simulink model "discrete_nonlinear_model"  (R2024a)
settings: Solver=ode45  StartTime=0.0  StopTime=10  RelTol=1e-3  EnableMultiTasking=on
values from neighbouring files (symbols this model uses):
  m = calculate_model(p, T, tau_e)    [init.m]
  omega0 = 20    [init.m]
  reg = syn_regulator(m, 0.1, T)    [init.m]
  T = 0.00064    [init.m]
  tau_e = 0.005    [init.m]
settings Model: Creator=oleg  LastModifiedBy=olgatsybina
settings SolverCC: AlgebraicLoopSolver=TrustRegion
settings DataIOCC: LimitDataPoints=on  SaveFormat=Array  ReturnWorkspaceOutputs=off
settings OptimizationCC: LifeSpan=inf
settings DebuggingCC: SolverPrmCheckMsg=warning  UnconnectedInputMsg=warning  UnconnectedOutputMsg=warning  UnconnectedLineMsg=warning  SFUnexpectedBacktrackingDiag=warning  SFNoUnconditionalDefaultTransitionDiag=warning  SFExecutionAtInitializationDiag=none  ArithmeticOperatorsInVariantConditions=warning
settings HardwareCC: ProdBitPerPointer=32  ProdBitPerSizeT=32  ProdBitPerPtrDiffT=32  ProdLargestAtomicFloat=None  ProdIntDivRoundTo=Undefined  ProdEndianess=Unspecified  ProdWordSize=32  ProdHWDeviceType=32-bit Generic
settings ModelReferenceCC: EnableRefExpFcnMdlSchedulingChecks=on  PropagateSignalLabelsOutOfModel=off
settings SFSimCC: SimUseLocalCustomCode=off  CustomCodeUndefinedFunction=UseInterfaceOnly
settings RTWCC: RTWUseLocalCustomCode=off  GPUComputeCapability=3.5  DLArmComputeVersion=19.05
settings CodeAppCC: StateflowObjectComments=on
settings GRTTargetCC: TargetLangStandard=C89/C90 (ANSI)
settings ConfigComp: CovMetricSettings=dw  CovSaveCumulativeToWorkspaceVar=on  CovSaveSingleToWorkspaceVar=on  CovExternalEMLEnable=off  CovSFcnEnable=off

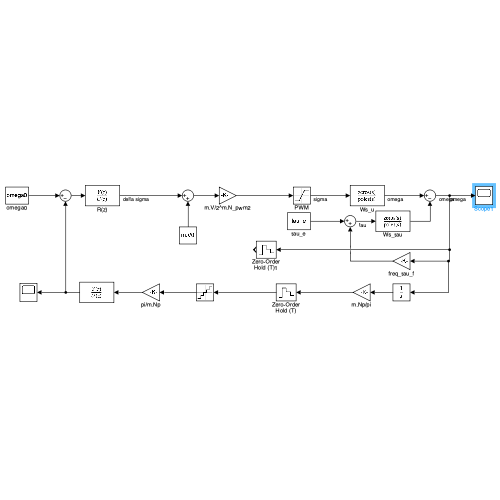
[thumbnail: Simulink's stored preview of the top-level diagram]
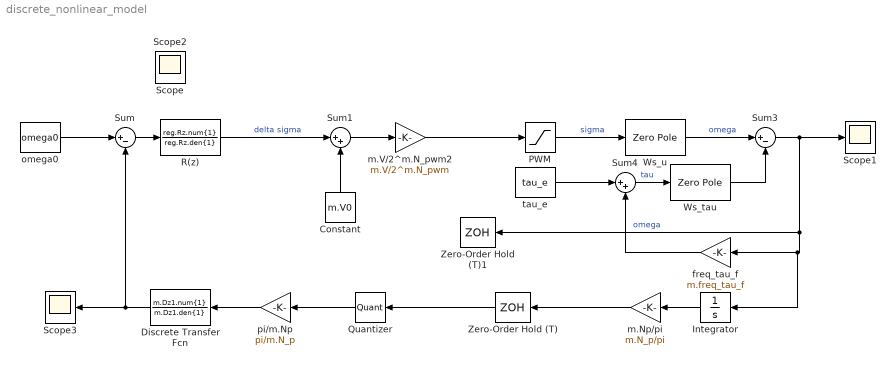
== system discrete_nonlinear_model ==
  Constant : Constant  Value=m.V0
  Discrete Transfer Fcn : DiscreteTransferFcn  Numerator=m.Dz1.num{1}  Denominator=m.Dz1.den{1}
  Integrator : Integrator
  PWM : Saturate  UpperLimit=m.V  LowerLimit=-m.V
  Quantizer : Quantizer  QuantizationInterval=1
  R(z) : DiscreteTransferFcn  Numerator=reg.Rz.num{1}  Denominator=reg.Rz.den{1}  SampleTime=T
  Scope{,1..3} (4 alike) : Scope
  Sum : Sum  Inputs=|+-
  Sum1 : Sum  Inputs=|++
  Sum3 : Sum  Inputs=|+-
  Sum4 : Sum  Inputs=|++
  Ws_tau : ZeroPole  Zeros=m.Ws_tau.Z{1}  Poles=m.Ws_tau.P{1}  Gain=m.Ws_tau.K
  Ws_u : ZeroPole  Zeros=m.Ws_u.Z{1}  Poles=m.Ws_u.P{1}  Gain=m.Ws_u.K
  Zero-Order Hold (T) : ZeroOrderHold  SampleTime=T
  Zero-Order Hold (T)1 : ZeroOrderHold  SampleTime=T
  freq_tau_f : Gain  Gain=m.freq_tau_f
  m.Np/pi : Gain  Gain=m.N_p/pi
  m.V/2^m.N_pwm2 : Gain  Gain=m.V/2^m.N_pwm
  omega0 : Constant  Value=omega0  SampleTime=T
  pi/m.Np : Gain  Gain=pi/m.N_p
  tau_e : Constant  Value=tau_e  SampleTime=T
  wires:
  omega0/1 -> Sum/1
  Sum/1 -> R(z)/1
  Zero-Order Hold (T)/1 -> Quantizer/1
  Sum3/1 -> Scope1/1, Zero-Order Hold (T)1/1, Integrator/1, freq_tau_f/1  "omega"
  freq_tau_f/1 -> Sum4/2
  Sum4/1 -> Ws_tau/1  "tau"
  tau_e/1 -> Sum4/1
  Ws_u/1 -> Sum3/1  "omega"
  Integrator/1 -> m.Np/pi/1
  m.Np/pi/1 -> Zero-Order Hold (T)/1
  R(z)/1 -> Sum1/1  "delta sigma"
  Quantizer/1 -> pi/m.Np/1
  Sum1/1 -> m.V/2^m.N_pwm2/1
  pi/m.Np/1 -> Discrete Transfer Fcn/1
  Discrete Transfer Fcn/1 -> Sum/2, Scope3/1
  m.V/2^m.N_pwm2/1 -> PWM/1
  PWM/1 -> Ws_u/1  "sigma"
  Constant/1 -> Sum1/2
  Ws_tau/1 -> Sum3/2
